simulink model "PassengerCar"  (R2019b)
settings: Solver=ode1  StartTime=0  StopTime=25  FixedStep=1.0000000000000000e-003  RelTol=1e-3
InitFcn:
  | sampleTime = str2double(get_param(bdroot, 'FixedStep'));
undefined symbols (not defined in the file or in its folder): AccPedalPos, BrakePedalPos, BrakeSwitch, DiscIntNeverNeededParam, DYNA4, EngSpd, IgnitionSwitch, InitialGear, InitialSpeed, IntendedEngTrq, LeftIndicator, MainBrakePress, MaxGear, MDL, MinGear, RefAcc, RefLane, RefLatPos, RefPath, RefPathCurv, RefSpd, RefSpdPreview, RefSpdRetrospect, RightIndicator, SteeringWheelAng, SteeringWheelTrq, UserDefinedRefValue, vm_const
libraries: UtilitiesLibrary x31, simulink x18, WheelSystemModules x13, LongitudinalControllerModules x13, LateralControllerModules x7, AnimationBusselectorModules x5, EnvironmentModules x5, BasicEngineControlModules x5, MiscellaneousControlModules x5, Animation3Modules x4, AuxiliariesModules x4, TireModules x4
(part 27 of 39)

== system PassengerCar/Vehicle/WheelSystem/RearRightWheelSystem/WheelOutput ==
  DriveBrakeTrq_wrt_WheelRotAxis(VehSys)[Nm]___UNIQUE_1 : Inport  Description=|  PortDimensions=[3]
      | <name>DriveBrakeTrq_wrt_WheelRotAxis(VehSys)[Nm]</name>
      | <comment></comment>
  RotSpd[rad/s]___UNIQUE_1 : Inport  Description=|  Port=2  PortDimensions=[1]
      | <name>RotSpd[rad/s]</name>
      | <comment></comment>
  RotAcc[rad/s**2]___UNIQUE_1 : Inport  Description=|  Port=3  PortDimensions=[1]
      | <name>RotAcc[rad/s**2]</name>
      | <comment></comment>
  BlockingState[0;1]___UNIQUE_1 : Inport  Description=|  Port=4  PortDimensions=[1]
      | <name>BlockingState[0;1]</name>
      | <comment></comment>
  RotAng[rad]___UNIQUE_1 : Inport  Description=|  Port=5  PortDimensions=[1]
      | <name>RotAng[rad]</name>
      | <comment></comment>
  BrakeTrqPressRatio[m**3]___UNIQUE_1 : Inport  Description=|  Port=6  PortDimensions=[1]
      | <name>BrakeTrqPressRatio[m**3]</name>
      | <comment></comment>
  RotAxisInrt[kg*m**2]___UNIQUE_1 : Inport  Description=|  Port=7  PortDimensions=[1]
      | <name>RotAxisInrt[kg*m**2]</name>
      | <comment></comment>
  TotalResistanceTorque[Nm]___UNIQUE_1 : Inport  Description=|  Port=8  PortDimensions=[1]
      | <name>TotalResistanceTorque[Nm]</name>
      | <comment></comment>
  KinematicWheelActiveFlag[0;1]___UNIQUE_1 : Inport  Description=|  Port=9  PortDimensions=[1]
      | <name>KinematicWheelActiveFlag[0;1]</name>
      | <comment></comment>
  VehBodyReplacementInrt[kg*m**2]___UNIQUE_1 : Inport  Description=|  Port=10  PortDimensions=[1]
      | <name>VehBodyReplacementInrt[kg*m**2]</name>
      | <comment></comment>
  __TDD__Wheel.BlockingState[0;1] : Demux  Outputs=[1]
  __TDD__Wheel.BrakeTrqPressRatio[m**3] : Demux  Outputs=[1]
  __TDD__Wheel.DriveBrakeTrq_wrt_WheelRotAxis(VehSys)[Nm] : Demux  Outputs=[3]
  __TDD__Wheel.KinematicWheelActiveFlag[0;1] : Demux  Outputs=[1]
  __TDD__Wheel.RotAcc[rad/s**2] : Demux  Outputs=[1]
  __TDD__Wheel.RotAng[rad] : Demux  Outputs=[1]
  __TDD__Wheel.RotAxisInrt[kg*m**2] : Demux  Outputs=[1]
  __TDD__Wheel.RotSpd[rad/s] : Demux  Outputs=[1]
  __TDD__Wheel.TotalResistanceTorque[Nm] : Demux  Outputs=[1]
  __TDD__Wheel.VehBodyReplacementInrt[kg*m**2] : Demux  Outputs=[1]
  __TDO__Wheel : BusCreator  Inputs=10
  Wheel___UNIQUE_1 : Outport  Description=|  PortDimensions=[12]  VectorParamsAs1DForOutWhenUnconnected=off
      | <name>DriveBrakeTrq_wrt_WheelRotAxis(VehSys)[Nm]</name>
      | <comment></comment>
  wires:
  DriveBrakeTrq_wrt_WheelRotAxis(VehSys)[Nm]___UNIQUE_1/1 -> __TDD__Wheel.DriveBrakeTrq_wrt_WheelRotAxis(VehSys)[Nm]/1
  __TDD__Wheel.DriveBrakeTrq_wrt_WheelRotAxis(VehSys)[Nm]/1 -> __TDO__Wheel/1  "DriveBrakeTrq_wrt_WheelRotAxis(VehSys)[Nm]"
  RotSpd[rad/s]___UNIQUE_1/1 -> __TDD__Wheel.RotSpd[rad/s]/1
  __TDD__Wheel.RotSpd[rad/s]/1 -> __TDO__Wheel/2  "RotSpd[rad/s]"
  RotAcc[rad/s**2]___UNIQUE_1/1 -> __TDD__Wheel.RotAcc[rad/s**2]/1
  __TDD__Wheel.RotAcc[rad/s**2]/1 -> __TDO__Wheel/3  "RotAcc[rad/s**2]"
  BlockingState[0;1]___UNIQUE_1/1 -> __TDD__Wheel.BlockingState[0;1]/1
  __TDD__Wheel.BlockingState[0;1]/1 -> __TDO__Wheel/4  "BlockingState[0;1]"
  RotAng[rad]___UNIQUE_1/1 -> __TDD__Wheel.RotAng[rad]/1
  __TDD__Wheel.RotAng[rad]/1 -> __TDO__Wheel/5  "RotAng[rad]"
  BrakeTrqPressRatio[m**3]___UNIQUE_1/1 -> __TDD__Wheel.BrakeTrqPressRatio[m**3]/1
  __TDD__Wheel.BrakeTrqPressRatio[m**3]/1 -> __TDO__Wheel/6  "BrakeTrqPressRatio[m**3]"
  RotAxisInrt[kg*m**2]___UNIQUE_1/1 -> __TDD__Wheel.RotAxisInrt[kg*m**2]/1
  __TDD__Wheel.RotAxisInrt[kg*m**2]/1 -> __TDO__Wheel/7  "RotAxisInrt[kg*m**2]"
  TotalResistanceTorque[Nm]___UNIQUE_1/1 -> __TDD__Wheel.TotalResistanceTorque[Nm]/1
  __TDD__Wheel.TotalResistanceTorque[Nm]/1 -> __TDO__Wheel/8  "TotalResistanceTorque[Nm]"
  KinematicWheelActiveFlag[0;1]___UNIQUE_1/1 -> __TDD__Wheel.KinematicWheelActiveFlag[0;1]/1
  __TDD__Wheel.KinematicWheelActiveFlag[0;1]/1 -> __TDO__Wheel/9  "KinematicWheelActiveFlag[0;1]"
  VehBodyReplacementInrt[kg*m**2]___UNIQUE_1/1 -> __TDD__Wheel.VehBodyReplacementInrt[kg*m**2]/1
  __TDD__Wheel.VehBodyReplacementInrt[kg*m**2]/1 -> __TDO__Wheel/10  "VehBodyReplacementInrt[kg*m**2]"
  __TDO__Wheel/1 -> Wheel___UNIQUE_1/1  "Wheel"

== system PassengerCar/Vehicle/WheelSystem/WheelSystemOutputs/FrontLeftOuput ==
  InnerTire___UNIQUE_1 : Inport  Description=|
      | <name>InnerTire</name>
      | <comment></comment>
  Tire___UNIQUE_1 : Inport  Description=|  Port=2
      | <name>Tire</name>
      | <comment></comment>
  Wheel___UNIQUE_1 : Inport  Description=|  Port=3
      | <name>Wheel</name>
      | <comment></comment>
  __TDO__FrontLeft : BusCreator  Inputs=3
  FrontLeft___UNIQUE_1 : Outport  Description=|  VectorParamsAs1DForOutWhenUnconnected=off
      | <name>InnerTire</name>
      | <comment></comment>
  wires:
  InnerTire___UNIQUE_1/1 -> __TDO__FrontLeft/1  "InnerTire"
  Tire___UNIQUE_1/1 -> __TDO__FrontLeft/2  "Tire"
  Wheel___UNIQUE_1/1 -> __TDO__FrontLeft/3  "Wheel"
  __TDO__FrontLeft/1 -> FrontLeft___UNIQUE_1/1  "FrontLeft"

== system PassengerCar/Vehicle/WheelSystem/WheelSystemOutputs/FrontRightOuput ==
  InnerTire___UNIQUE_1 : Inport  Description=|
      | <name>InnerTire</name>
      | <comment></comment>
  Tire___UNIQUE_1 : Inport  Description=|  Port=2
      | <name>Tire</name>
      | <comment></comment>
  Wheel___UNIQUE_1 : Inport  Description=|  Port=3
      | <name>Wheel</name>
      | <comment></comment>
  __TDO__FrontRight : BusCreator  Inputs=3
  FrontRight___UNIQUE_1 : Outport  Description=|  VectorParamsAs1DForOutWhenUnconnected=off
      | <name>InnerTire</name>
      | <comment></comment>
  wires:
  InnerTire___UNIQUE_1/1 -> __TDO__FrontRight/1  "InnerTire"
  Tire___UNIQUE_1/1 -> __TDO__FrontRight/2  "Tire"
  Wheel___UNIQUE_1/1 -> __TDO__FrontRight/3  "Wheel"
  __TDO__FrontRight/1 -> FrontRight___UNIQUE_1/1  "FrontRight"

== system PassengerCar/Vehicle/WheelSystem/WheelSystemOutputs/Rear2LeftOuput ==
  InnerTire___UNIQUE_1 : Inport  Description=|
      | <name>InnerTire</name>
      | <comment></comment>
  Tire___UNIQUE_1 : Inport  Description=|  Port=2
      | <name>Tire</name>
      | <comment></comment>
  Wheel___UNIQUE_1 : Inport  Description=|  Port=3
      | <name>Wheel</name>
      | <comment></comment>
  __TDO__Rear2Left : BusCreator  Inputs=3
  Rear2Left___UNIQUE_1 : Outport  Description=|  VectorParamsAs1DForOutWhenUnconnected=off
      | <name>InnerTire</name>
      | <comment></comment>
  wires:
  InnerTire___UNIQUE_1/1 -> __TDO__Rear2Left/1  "InnerTire"
  Tire___UNIQUE_1/1 -> __TDO__Rear2Left/2  "Tire"
  Wheel___UNIQUE_1/1 -> __TDO__Rear2Left/3  "Wheel"
  __TDO__Rear2Left/1 -> Rear2Left___UNIQUE_1/1  "Rear2Left"

== system PassengerCar/Vehicle/WheelSystem/WheelSystemOutputs/Rear2RightOuput ==
  InnerTire___UNIQUE_1 : Inport  Description=|
      | <name>InnerTire</name>
      | <comment></comment>
  Tire___UNIQUE_1 : Inport  Description=|  Port=2
      | <name>Tire</name>
      | <comment></comment>
  Wheel___UNIQUE_1 : Inport  Description=|  Port=3
      | <name>Wheel</name>
      | <comment></comment>
  __TDO__Rear2Right : BusCreator  Inputs=3
  Rear2Right___UNIQUE_1 : Outport  Description=|  VectorParamsAs1DForOutWhenUnconnected=off
      | <name>InnerTire</name>
      | <comment></comment>
  wires:
  InnerTire___UNIQUE_1/1 -> __TDO__Rear2Right/1  "InnerTire"
  Tire___UNIQUE_1/1 -> __TDO__Rear2Right/2  "Tire"
  Wheel___UNIQUE_1/1 -> __TDO__Rear2Right/3  "Wheel"
  __TDO__Rear2Right/1 -> Rear2Right___UNIQUE_1/1  "Rear2Right"

== system PassengerCar/Vehicle/WheelSystem/WheelSystemOutputs/Rear3LeftOuput ==
  InnerTire___UNIQUE_1 : Inport  Description=|
      | <name>InnerTire</name>
      | <comment></comment>
  Tire___UNIQUE_1 : Inport  Description=|  Port=2
      | <name>Tire</name>
      | <comment></comment>
  Wheel___UNIQUE_1 : Inport  Description=|  Port=3
      | <name>Wheel</name>
      | <comment></comment>
  __TDO__Rear3Left : BusCreator  Inputs=3
  Rear3Left___UNIQUE_1 : Outport  Description=|  VectorParamsAs1DForOutWhenUnconnected=off
      | <name>InnerTire</name>
      | <comment></comment>
  wires:
  InnerTire___UNIQUE_1/1 -> __TDO__Rear3Left/1  "InnerTire"
  Tire___UNIQUE_1/1 -> __TDO__Rear3Left/2  "Tire"
  Wheel___UNIQUE_1/1 -> __TDO__Rear3Left/3  "Wheel"
  __TDO__Rear3Left/1 -> Rear3Left___UNIQUE_1/1  "Rear3Left"

== system PassengerCar/Vehicle/WheelSystem/WheelSystemOutputs/Rear3RightOuput ==
  InnerTire___UNIQUE_1 : Inport  Description=|
      | <name>InnerTire</name>
      | <comment></comment>
  Tire___UNIQUE_1 : Inport  Description=|  Port=2
      | <name>Tire</name>
      | <comment></comment>
  Wheel___UNIQUE_1 : Inport  Description=|  Port=3
      | <name>Wheel</name>
      | <comment></comment>
  __TDO__Rear3Right : BusCreator  Inputs=3
  Rear3Right___UNIQUE_1 : Outport  Description=|  VectorParamsAs1DForOutWhenUnconnected=off
      | <name>InnerTire</name>
      | <comment></comment>
  wires:
  InnerTire___UNIQUE_1/1 -> __TDO__Rear3Right/1  "InnerTire"
  Tire___UNIQUE_1/1 -> __TDO__Rear3Right/2  "Tire"
  Wheel___UNIQUE_1/1 -> __TDO__Rear3Right/3  "Wheel"
  __TDO__Rear3Right/1 -> Rear3Right___UNIQUE_1/1  "Rear3Right"

== system PassengerCar/Vehicle/WheelSystem/WheelSystemOutputs/RearLeftOuput ==
  InnerTire___UNIQUE_1 : Inport  Description=|
      | <name>InnerTire</name>
      | <comment></comment>
  Tire___UNIQUE_1 : Inport  Description=|  Port=2
      | <name>Tire</name>
      | <comment></comment>
  Wheel___UNIQUE_1 : Inport  Description=|  Port=3
      | <name>Wheel</name>
      | <comment></comment>
  __TDO__RearLeft : BusCreator  Inputs=3
  RearLeft___UNIQUE_1 : Outport  Description=|  VectorParamsAs1DForOutWhenUnconnected=off
      | <name>InnerTire</name>
      | <comment></comment>
  wires:
  InnerTire___UNIQUE_1/1 -> __TDO__RearLeft/1  "InnerTire"
  Tire___UNIQUE_1/1 -> __TDO__RearLeft/2  "Tire"
  Wheel___UNIQUE_1/1 -> __TDO__RearLeft/3  "Wheel"
  __TDO__RearLeft/1 -> RearLeft___UNIQUE_1/1  "RearLeft"

== system PassengerCar/Vehicle/WheelSystem/WheelSystemOutputs/RearRightOuput ==
  InnerTire___UNIQUE_1 : Inport  Description=|
      | <name>InnerTire</name>
      | <comment></comment>
  Tire___UNIQUE_1 : Inport  Description=|  Port=2
      | <name>Tire</name>
      | <comment></comment>
  Wheel___UNIQUE_1 : Inport  Description=|  Port=3
      | <name>Wheel</name>
      | <comment></comment>
  __TDO__RearRight : BusCreator  Inputs=3
  RearRight___UNIQUE_1 : Outport  Description=|  VectorParamsAs1DForOutWhenUnconnected=off
      | <name>InnerTire</name>
      | <comment></comment>
  wires:
  InnerTire___UNIQUE_1/1 -> __TDO__RearRight/1  "InnerTire"
  Tire___UNIQUE_1/1 -> __TDO__RearRight/2  "Tire"
  Wheel___UNIQUE_1/1 -> __TDO__RearRight/3  "Wheel"
  __TDO__RearRight/1 -> RearRight___UNIQUE_1/1  "RearRight"

== system PassengerCar/Vehicle/WheelSystem/WheelSystemOutputs/WheelSystemOutput ==
  FrontLeft___UNIQUE_1 : Inport  Description=|
      | <name>FrontLeft</name>
      | <comment></comment>
  FrontRight___UNIQUE_1 : Inport  Description=|  Port=2
      | <name>FrontRight</name>
      | <comment></comment>
  RearLeft___UNIQUE_1 : Inport  Description=|  Port=3
      | <name>RearLeft</name>
      | <comment></comment>
  RearRight___UNIQUE_1 : Inport  Description=|  Port=4
      | <name>RearRight</name>
      | <comment></comment>
  Rear2Left___UNIQUE_1 : Inport  Description=|  Port=5
      | <name>Rear2Left</name>
      | <comment></comment>
  Rear2Right___UNIQUE_1 : Inport  Description=|  Port=6
      | <name>Rear2Right</name>
      | <comment></comment>
  Rear3Left___UNIQUE_1 : Inport  Description=|  Port=7
      | <name>Rear3Left</name>
      | <comment></comment>
  Rear3Right___UNIQUE_1 : Inport  Description=|  Port=8
      | <name>Rear3Right</name>
      | <comment></comment>
  __TDO__WheelSystem : BusCreator  Inputs=8
  WheelSystem___UNIQUE_1 : Outport  Description=|  VectorParamsAs1DForOutWhenUnconnected=off
      | <name>FrontLeft</name>
      | <comment></comment>
  wires:
  FrontLeft___UNIQUE_1/1 -> __TDO__WheelSystem/1  "FrontLeft"
  FrontRight___UNIQUE_1/1 -> __TDO__WheelSystem/2  "FrontRight"
  RearLeft___UNIQUE_1/1 -> __TDO__WheelSystem/3  "RearLeft"
  RearRight___UNIQUE_1/1 -> __TDO__WheelSystem/4  "RearRight"
  Rear2Left___UNIQUE_1/1 -> __TDO__WheelSystem/5  "Rear2Left"
  Rear2Right___UNIQUE_1/1 -> __TDO__WheelSystem/6  "Rear2Right"
  Rear3Left___UNIQUE_1/1 -> __TDO__WheelSystem/7  "Rear3Left"
  Rear3Right___UNIQUE_1/1 -> __TDO__WheelSystem/8  "Rear3Right"
  __TDO__WheelSystem/1 -> WheelSystem___UNIQUE_1/1  "WheelSystem"

== system PassengerCar/VehicleControl/LateralControl/Disabled LateralControl/ControlSystems ==
  note: How to add user-defined lateral additional inputs to the model:
      |
      | 1. Open the block "LateralControlOutput" by double-clicking on it.
      | 2. Edit the signals "UserDefined.<signalname>" inside by renaming them and setting the unit. You can also add signals to the existing ones.
      | Be careful to always use the prefix "UserDefined." for additional signals!!!
      | 4. Save the model to apply your changes.
  Control Systems Parameters : Subsystem
  DynaSystemInfo : Subsystem  Tag=DynaSystemInfo
      mask init:
      | data = get_param(gcb, 'UserData');
      settings: OpenFcn=DYNA4.ModelHandling.System.ShowEditSystemInformationDialog(gcb);
      mask Display: disp(['Type = ', data.type, '\nName = ', data.name ])
  Lateral Controller : Subsystem
  LateralControlOutput : Subsystem  Tag=TESIS DYNAware Interface Block  mask{NeedsUpdate=off}
      mask prompts: NeedsUpdate "Specify, if subsystem content needs to be updated"
      mask help: DYNA4 Interface Block Version 4.2
      mask init:
      | blockName = get_param(gcbh, 'Name');
      | parentId = DYNA4.ModelHandling.AccessID.getFromHierarchy(gcbh);
      | TD.InterfaceBlock.ModelCallbacks.GenerateContent(gcb);
      settings: AttributesFormatString=(Grounded Input)  DeleteFcn=TD.InterfaceBlock.ModelCallbacks.CloseGUI( gcbh );  NameChangeFcn=TD.InterfaceBlock.ModelCallbacks.BlockRenamedHandler(gcbh);  OpenFcn=TD.InterfaceBlock.ModelCallbacks.OpenGUI( gcbh );  CloseFcn=TD.InterfaceBlock.ModelCallbacks.CloseGUI( gcbh );
      mask Display:
      | image('dm_intfblk_lib.jpg','center');
      | port_label('output',1, 'LateralControl');
  LateralControl : Outport  VectorParamsAs1DForOutWhenUnconnected=off
  wires:
  LateralControlOutput/1(LateralControl___UNIQUE_1) -> LateralControl/1

== system PassengerCar/VehicleControl/LateralControl/Disabled LateralControl/ControlSystemsPreprocessor ==
  Maneuver : Subsystem
      settings: CopyFcn=DYNA4.Internal.ModelCallbacks.Modules.UpdateMaskParameters(gcb);  NameChangeFcn=DYNA4.Internal.ModelCallbacks.Modules.UpdateMaskParameters(gcb);

== system PassengerCar/VehicleControl/LateralControl/Disabled LateralControl/DynaSystemInfo ==

== system PassengerCar/VehicleControl/LateralControl/Enabled LateralControl/ControlSystems ==
  note: How to add user-defined lateral additional inputs to the model:
      |
      | 1. Open the block "LateralControlOutput" by double-clicking on it.
      | 2. Edit the signals "UserDefined.<signalname>" inside by renaming them and setting the unit. You can also add signals to the existing ones.
      | Be careful to always use the prefix "UserDefined." for additional signals!!!
      | 3. Adjust the size of the demux-block of the user-defined signals on the left of the bus-creator so that all ports can be connected.
      | 4. Save the model to apply your changes.
  Phase[-] : Inport
  TaskIdentifiers : Inport  Port=2
  SourceIdentifiers : Inport  Port=3
  ControlInputs : Inport  Port=4
  UserDefinedSignals : Inport  Port=5
  VehicleInfo : Inport  Port=6
  CtrlSystemsAbscissae : Inport  Port=7
  Bus Selector1 : BusSelector  OutputSignals=SteeringWheelTrq[Nm],SteeringWheelInputSwitch[-]
  Bus Selector2 : BusSelector  OutputSignals=LeftIndicator,RightIndicator
  Control Systems Parameters : Subsystem
  Demux : Demux  Outputs=2
  DynaSystemInfo : Subsystem  Tag=DynaSystemInfo
      mask init:
      | data = get_param(gcb, 'UserData');
      settings: OpenFcn=DYNA4.ModelHandling.System.ShowEditSystemInformationDialog(gcb);
      mask Display: disp(['Type = ', data.type, '\nName = ', data.name ])
  Lateral Controller : Subsystem
  LateralControlOutput : Subsystem  Tag=TESIS DYNAware Interface Block  mask{NeedsUpdate=off, SignalInfo=|}
      mask SignalInfo=|
      | {
      |   "Version": "4.6",
      |   "MuxedOutputBusName": "LateralControl",
      |   "MuxedInputBusName": "fromCTRL",
      |   "MuxedInputSelected": false,
      |   "MuxedOutputSelected": true,
      |   "SignalData": [
      |     {
      |       "initialValue": "0.0",
      |       "name": "SteeringWheelAng[rad]",
      |       "comment": "Steering wheel angle",
      |       "minString": "",
      |       "maxString": "",
      |       "width": 1,
      |       "dataType": 0,
      |       "signalType": 0,
      |       "createSignal": false,
      |       "outputName": "SteeringWheelAng[rad]",
      |       "generateSignalAccessBlock": false,
      |       "accessId": "$(parentId).$(blockName).$(outputName)"
      |     },
      |     {
      |       "initialValue": "0.0",
      |       "name": "SteeringWheelTrq[Nm]",
      |       "comment": "Steering wheel torque",
      |       "minString": "",
      |       "maxString": "",
      |       "width": 1,
      |       "dataType": 0,
      |       "signalType": 0,
      |       "createSignal": false,
      |       "outputName": "SteeringWheelTrq[Nm]",
      |       "generateSignalAccessBlock": false,
      |       "accessId": "$(parentId).$(blockName).$(outputName)"
      |     },
      |     {
      |       "initialValue": "0.0",
      |       "name": "SteeringWheelInputSwitch[-]",
      |       "comment": "Steering wheel input switch (0: angle, 1: torque)",
      |       "minString": "",
      |       "maxString": "",
      |       "width": 1,
      |       "dataType": 0,
      |       "signalType": 0,
      |       "createSignal": false,
      |       "outputName": "SteeringWheelInputSwitch[-]",
      |       "generateSignalAccessBlock": false,
      |       "accessId": "$(parentId).$(blockName).$(outputName)"
      |     },
      |     {
      |       "initialValue": "0.0",
      |       "name": "UserDefinedRefValue[-]",
      |       "comment": "User-defined reference value",
      |       "minString": "",
      |       "maxString": "",
      |       "width": 1,
      |       "dataType": 0,
      |       "signalType": 0,
      |       "createSignal": false,
      |       "outputName": "UserDefinedRefValue[-]",
      |       "generateSignalAccessBlock": false,
      |       "accessId": "$(parentId).$(blockName).$(outputName)"
      |     },
      |     {
      |       "initialValue": "0.0",
      |       "name": "LeftIndicator[0;1]",
      |       "comment": "Left indicator state",
      |       "minString": "",
      |       "maxString": "",
      |       "width": 1,
      |       "dataType": 0,
      |       "signalType": 0,
      |       "createSignal": false,
      |       "outputName": "LeftIndicator[0;1]",
      |       "generateSignalAccessBlock": false,
      |       "accessId": "$(parentId).$(blockName).$(outputName)"
      |     },
      |     {
      |       "initialValue": "0.0",
      |       "name": "RightIndicator[0;1]",
      |       "comment": "Right indicator state",
      |       "minString": "",
      |       "maxString": "",
      |       "width": 1,
      |       "dataType": 0,
      |       "signalType": 0,
      |       "createSignal": false,
      |       "outputName": "RightIndicator[0;1]",
      |       "generateSignalAccessBlock": false,
      |       "accessId": "$(parentId).$(blockName).$(outputName)"
      |     },
      |     {
      |       "initialValue": "0.0",
      |       "name": "LateralPhase[-]",
      |       "comment": "Lateral phase number",
      |       "minString": "",
      |       "maxString": "",
      |       "width": 1,
      |       "dataType": 0,
      |       "signalType": 0,
      |       "createSignal": false,
      |       "outputName": "LateralPhase[-]",
      |       "generateSignalAccessBlock": false,
      |       "accessId": "$(parentId).$(blockName).$(outputName)"
      |     },
      |     {
      |       "initialValue": "0.0",
      |       "name": "UserDefined.UserDefined1[-]",
      |       "comment": "User-defined additional input 1 (can be edited by the user)",
      |       "minString": "",
      |       "maxString": "",
      |       "width": 1,
      |       "dataType": 0,
      |       "signalType": 0,
      |       "createSignal": false,
      |       "outputName": "UserDefined1[-]",
      |       "generateSignalAccessBlock": false,
      |       "accessId": "$(parentId).$(blockName).$(outputName)"
      |     },
      |     {
      |       "initialValue": "0.0",
      |       "name": "UserDefined.UserDefined2[-]",
      |       "comment": "User-defined additional input 2 (can be edited by the user)",
      |       "minString": "",
      |       "maxString": "",
      |       "width": 1,
      |       "dataType": 0,
      |       "signalType": 0,
      |       "createSignal": false,
      |       "outputName": "UserDefined2[-]",
      |       "generateSignalAccessBlock": false,
      |       "accessId": "$(parentId).$(blockName).$(outputName)"
      |     }
      |   ]
      | }
      mask prompts: NeedsUpdate "Specify, if subsystem content needs to be updated"; SignalInfo "Signal Info (json)"
      mask help: DYNA4 Interface Block Version 4.6
      mask init:
      | blockName = get_param(gcbh, 'Name');
      | parentId = DYNA4.ModelHandling.AccessID.getFromHierarchy(gcbh);
      | TD.InterfaceBlock.ModelCallbacks.GenerateContent(gcb);
      settings: DeleteFcn=TD.InterfaceBlock.ModelCallbacks.CloseGUI( gcbh );  NameChangeFcn=TD.InterfaceBlock.ModelCallbacks.BlockRenamedHandler(gcbh);  OpenFcn=TD.InterfaceBlock.ModelCallbacks.OpenGUI( gcbh );  CloseFcn=TD.InterfaceBlock.ModelCallbacks.CloseGUI( gcbh );
      mask Display:
      | image('InterfaceBlock.png','center');
      | port_label('input',1, 'SteeringWheelAng[rad]');
      | port_label('input',2, 'SteeringWheelTrq[Nm]');
      | port_label('input',3, 'SteeringWheelInputSwitch[-]');
      | port_label('input',4, 'UserDefinedRefValue[-]');
      | port_label('input',5, 'LeftIndicator[0;1]');
      | port_label('input',6, 'RightIndicator[0;1]');
      | port_label('input',7, 'LateralPhase[-]');
      | port_label('input',8, 'UserDefined.UserDefined1[-]');
      | port_label('input',9, 'UserDefined.UserDefined2[-]');
      | port_label('output',1, 'LateralControl');
  SteeringWheelLimitation : Subsystem
  LateralControl : Outport  VectorParamsAs1DForOutWhenUnconnected=off
  ControllerParameters : Outport  Port=2  VectorParamsAs1DForOutWhenUnconnected=off
  wires:
  Phase[-]/1 -> LateralControlOutput/7(LateralPhase[-]___UNIQUE_1)
  Bus Selector1/1 -> LateralControlOutput/2(SteeringWheelTrq[Nm]___UNIQUE_1)  "<SteeringWheelTrq[Nm]>"
  Bus Selector1/2 -> LateralControlOutput/3(SteeringWheelInputSwitch[-]___UNIQUE_1)  "<SteeringWheelInputSwitch[-]>"
  UserDefinedSignals/1 -> Demux/1
  Control Systems Parameters/1(ControllerParameters) -> ControllerParameters/1, Lateral Controller/4(ControllerParameters)
  Demux/2 -> LateralControlOutput/9(UserDefined2[-]___UNIQUE_1)
  Demux/1 -> LateralControlOutput/8(UserDefined1[-]___UNIQUE_1)
  CtrlSystemsAbscissae/1 -> Control Systems Parameters/2(CtrlSystemsAbscissae)
  SteeringWheelLimitation/1(ModifiedSteeringWhlAng[rad]) -> LateralControlOutput/1(SteeringWheelAng[rad]___UNIQUE_1)
  ControlInputs/1 -> Lateral Controller/3(ControlInputs), SteeringWheelLimitation/2(ControlInputs), Bus Selector2/1
  Lateral Controller/1(SteeringWheelDemands) -> SteeringWheelLimitation/1(SteeringWheelDemands), Bus Selector1/1
  Bus Selector2/2 -> LateralControlOutput/6(RightIndicator[0;1]___UNIQUE_1)  "<RightIndicator>"
  Lateral Controller/2(UserDefinedRefValue[-]) -> LateralControlOutput/4(UserDefinedRefValue[-]___UNIQUE_1)
  TaskIdentifiers/1 -> Lateral Controller/1(TaskIdentifiers), Control Systems Parameters/1(TaskIdentifier)
  Bus Selector2/1 -> LateralControlOutput/5(LeftIndicator[0;1]___UNIQUE_1)  "<LeftIndicator>"
  VehicleInfo/1 -> Lateral Controller/5(VehicleInfo)
  SourceIdentifiers/1 -> Lateral Controller/2(SourceIdentifiers)
  LateralControlOutput/1(LateralControl___UNIQUE_1) -> LateralControl/1

== system PassengerCar/VehicleControl/LateralControl/Enabled LateralControl/ControlSystemsPreprocessor ==
  SchedulerAbscissae : Inport
  PhaseTerminationVals : Inport  Port=2
  LatCTRL : Inport  Port=3
  ExtCtrlVariablesEnforced : Inport  Port=4
  ExtCtrlVals : Inport  Port=5
  ControllerParameters : Inport  Port=6
  VehicleInfo : Inport  Port=7
  "External Presetting of Controller " : Subsystem
  Generation of Guidance Data : Subsystem
  Generation of Hold Data : Subsystem
  Maneuver : ManeuverControlModules/LateralManeuver  DATA_NODE=MDL.VehicleControl.LateralControl.Maneuver  Scheduler=MDL.VehicleControl.LateralControl.Maneuver.Scheduler
  Switch between Data Sources : Subsystem
  Phase[-] : Outport  VectorParamsAs1DForOutWhenUnconnected=off
  TaskIdentifiers : Outport  Port=2  VectorParamsAs1DForOutWhenUnconnected=off
  SourceIdentifiers : Outport  Port=3  VectorParamsAs1DForOutWhenUnconnected=off
  ControlInputs : Outport  Port=4  VectorParamsAs1DForOutWhenUnconnected=off
  UserDefinedSignals : Outport  Port=5  VectorParamsAs1DForOutWhenUnconnected=off
  wires:
  Maneuver/1 -> Phase[-]/1
  Maneuver/6 -> UserDefinedSignals/1
  LatCTRL/1 -> Generation of Hold Data/2(LatCTRL)
  Switch between Data Sources/1(SwitchedControlInputs) -> Generation of Guidance Data/2(ControlInputs)
  Generation of Guidance Data/1(ExtendedControlInputs) -> ControlInputs/1
  "External Presetting of Controller "/2(ModifiedSourceIdentifiers) -> Switch between Data Sources/1(SourceIdentifiers), SourceIdentifiers/1
  "External Presetting of Controller "/1(ModifiedTaskIdentifiers) -> Generation of Guidance Data/1(TaskIdentifiers), TaskIdentifiers/1
  ExtCtrlVariablesEnforced/1 -> "External Presetting of Controller "/3(ExtCtrlVariablesEnforced)
  SchedulerAbscissae/1 -> Maneuver/1
  PhaseTerminationVals/1 -> Maneuver/2
  Maneuver/2 -> Generation of Hold Data/1(PhaseTrigger)
  Maneuver/4 -> "External Presetting of Controller "/2(SourceIdentifiers)
  Maneuver/3 -> "External Presetting of Controller "/1(TaskIdentifiers)
  VehicleInfo/1 -> Generation of Guidance Data/4(VehicleInfo), Generation of Hold Data/3(VehicleInfo)
  ControllerParameters/1 -> Generation of Guidance Data/3(ControllerParameters)
  Maneuver/5 -> Switch between Data Sources/2(ControlInputs)
  Generation of Hold Data/1(HoldData) -> Switch between Data Sources/3(HoldData)
  ExtCtrlVals/1 -> Switch between Data Sources/4(ExternalData)

== system PassengerCar/VehicleControl/LateralControl/Enabled LateralControl/DynaSystemInfo ==

== system PassengerCar/VehicleControl/LongitudinalControl/ControlSystems/Brake System Switch and Pedal Limitation ==
  note: TASK_LONG_ACC_BRAKE_INPUTS = 1;
      | 	TASK_LONG_SPEED_CONTROL = 2;
      | 	TASK_LONG_ACCELERATION_CONTROL = 3;
      | 	TASK_LONG_USER_DEFINED = 4;
  note: SUBTASK_LONG_ACC_BRAKEPEDAL = 1;
      | 	SUBTASK_LONG_ACC_BRAKEPRESSURE_MAIN = 2;
      | 	SUBTASK_LONG_ACC_BRAKEPRESSURES = 3;
  ControlOutputs : Inport
  TaskIdentifiers : Inport  Port=2
  VehicleInfoSpeedControl : Inport  Port=3
  ControlInputs : Inport  Port=4
  AccBrakeLimitation : Subsystem
  BrakeSwitch = 1 : Subsystem  TreatAsAtomicUnit=on
  BrakeSwitch = 2 : Subsystem  TreatAsAtomicUnit=on
  Bus Assignment : BusAssignment  AssignedSignals=BrakeSwitch,AccPedalPos,BrakePedalPos,MainBrakePress
  Bus Selector : BusSelector  OutputSignals=VehicleDriverInfo_MaxMainBrakePress[Pa]
  Bus Selector1 : BusSelector  OutputSignals=AccPedalPos,BrakePedalPos,MainBrakePress
  Bus Selector2 : BusSelector  OutputSignals=BrakePedalPos,MainBrakePressure
  Bus Selector4 : BusSelector  OutputSignals=FrontLeftWheelBrakePress,FrontRightWheelBrakePress,RearLeftWheelBrakePress,RearRightWheelBrakePress,Rear2LeftWheelBrakePress,Rear2RightWheelBrakePress,Rear3LeftWheelBrakePress,Rear3RightWheelBrakePress,TrailerFrontLeftWheelBrakePress,TrailerFrontRightWheelBrakePress,TrailerRearLeftWheelBrakePress,TrailerRearRightWheelBrakePress,TrailerRear2LeftWheelBrakePress,TrailerRear2RightWheelBrakePress,TrailerRear3LeftWheelBrakePress,TrailerRear3RightWheelBrakePress  OutputAsBus=on
  Bus Selector7 : BusSelector  OutputSignals=Task,Subtask
  Constant : Constant  Value=vm_const('SUBTASK_LONG_ACC_BRAKEPEDAL')
  "Constant, Table, Automatic, Sine4" : simulink/Logic and Bit Operations/Compare To Constant  relop=~=  const=vm_const('TASK_LONG_ACC_BRAKE_INPUTS')  OutDataTypeStr=uint8  ZeroCross=off
  Default : Subsystem  TreatAsAtomicUnit=on
  Merge : Merge  Inputs=3
  Switch : Switch  Criteria=u2 > Threshold
  Switch Case : SwitchCase  CaseConditions={1, 2}
  ModifiedControlOutputs : Outport  VectorParamsAs1DForOutWhenUnconnected=off
  wires:
  ControlOutputs/1 -> Bus Selector4/1, Bus Selector1/1, Bus Assignment/1
  VehicleInfoSpeedControl/1 -> Bus Selector/1
  Switch/1 -> Switch Case/1, Bus Assignment/2  "BrakeSwitch[-]"
  Bus Selector7/2 -> Switch/3  "<Subtask>"
  Constant/1 -> Switch/1
  "Constant, Table, Automatic, Sine4"/1 -> Switch/2
  Bus Selector7/1 -> "Constant, Table, Automatic, Sine4"/1  "<Task>"
  TaskIdentifiers/1 -> Bus Selector7/1
  Switch Case/1 -> BrakeSwitch = 1/Action
  Switch Case/2 -> BrakeSwitch = 2/Action
  Switch Case/3 -> Default/Action
  Merge/1 -> Bus Selector2/1
  Bus Selector1/2 -> BrakeSwitch = 1/1(BrakePedalPos)  "<BrakePedalPos>"
  Bus Assignment/1 -> ModifiedControlOutputs/1
  Bus Selector/1 -> BrakeSwitch = 2/2(MaxMainBrakePressure), Default/2(MaxMainBrakePressure)  "<VehicleDriverInfo_MaxMainBrakePress[Pa]>"
  Bus Selector4/1 -> BrakeSwitch = 1/2(WheelBrakePressures), Default/1(WheelBrakePressures)
  Bus Selector1/3 -> BrakeSwitch = 2/1(MainBrakePressure)  "<MainBrakePress>"
  BrakeSwitch = 1/1(BrakeOutput) -> Merge/1
  BrakeSwitch = 2/1(BrakeOutput) -> Merge/2
  Default/1(BrakeOutput) -> Merge/3
  ControlInputs/1 -> AccBrakeLimitation/3(ControlInputs)
  Bus Selector2/2 -> Bus Assignment/5  "<MainBrakePressure>"
  Bus Selector2/1 -> AccBrakeLimitation/2(BrakePedalPos[0_1])  "<BrakePedalPos>"
  AccBrakeLimitation/1(AccPedalPosLimited) -> Bus Assignment/3
  AccBrakeLimitation/2(BrakePedalPosLimited) -> Bus Assignment/4
  Bus Selector1/1 -> AccBrakeLimitation/1(AccPedalPos[0_1])  "<AccPedalPos>"
